simulink model "quietdriverMV"  (R2024b)
settings: Solver=VariableStepAuto  StartTime=0.0  StopTime=100  RelTol=1e-3
libraries: simulink x1
settings Model: Creator=sprinkle
settings OptimizationCC: ReuseModelBlockBuffer=off
settings RTWCC: GPUComputeCapability=3.5

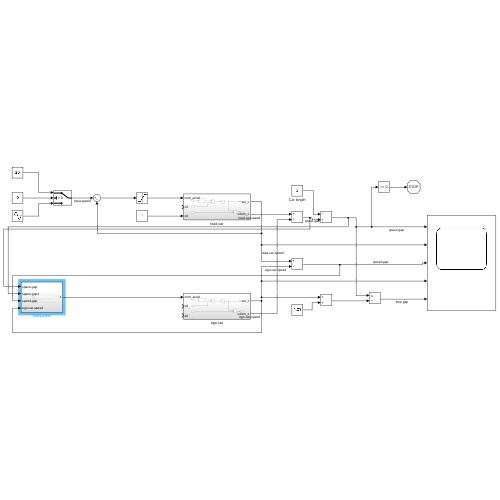
[thumbnail: Simulink's stored preview of the top-level diagram]
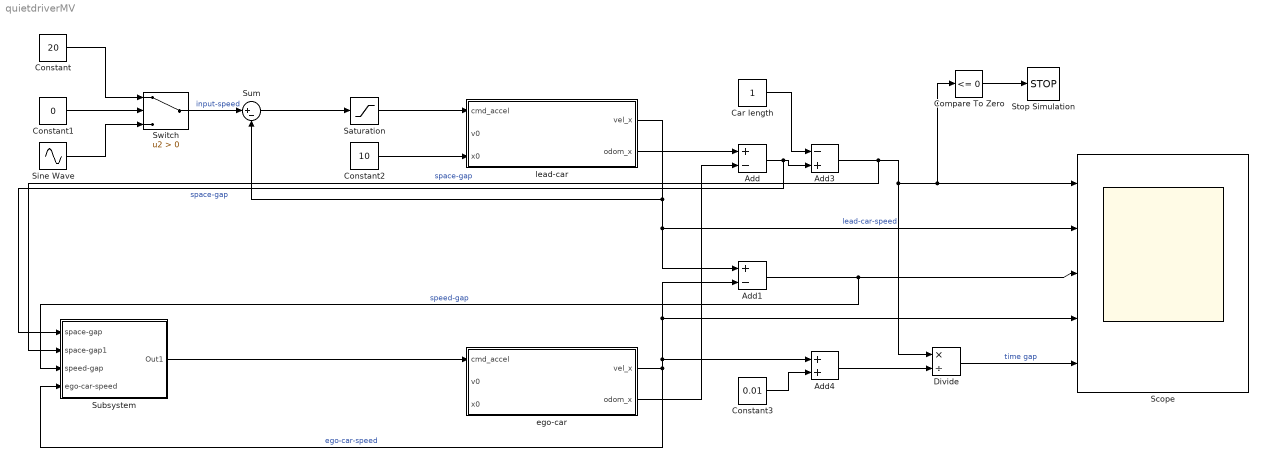
== system quietdriverMV ==
  Add : Sum  Inputs=+-
  Add1 : Sum  Inputs=+-
  Add3 : Sum  Inputs=-+
  Add4 : Sum
  Car length : Constant
  Compare To Zero : simulink/Logic and Bit Operations/Compare To Zero  relop=<=  OutDataTypeStr=boolean
  Constant : Constant  Value=20
  Constant1 : Constant  Value=0
  Constant2 : Constant  Value=10
  Constant3 : Constant  Value=0.01
  Divide : Product  Inputs=*/
  Saturation : Saturate  UpperLimit=1.5  LowerLimit=-3
  Scope : Scope  NumInputPorts=5
  Sine Wave : Sin  Bias=20  SampleTime=0
  Stop Simulation : Stop
  Subsystem : Subsystem
  Sum : Sum  Inputs=|+-
  Switch : Switch  Criteria=u2 > Threshold  SaturateOnIntegerOverflow=off  InputSameDT=off
  ego-car : Subsystem
  lead-car : Subsystem
  wires:
  Constant/1 -> Switch/1
  Sum/1 -> Saturation/1
  lead-car/1(vel_x) -> Add1/1, Scope/2, Sum/2  "lead-car-speed"
  Saturation/1 -> lead-car/1(cmd_accel)
  Switch/1 -> Sum/1  "input-speed"
  Sine Wave/1 -> Switch/3
  Constant1/1 -> Switch/2
  ego-car/1(vel_x) -> Subsystem/4(ego-car-speed), Add1/2, Scope/4, Add4/1  "ego-car-speed"
  lead-car/2(odom_x) -> Add/1
  ego-car/2(odom_x) -> Add/2
  Add3/1 -> Subsystem/2(space-gap1), Divide/1, Compare To Zero/1, Scope/1  "space-gap"
  Add1/1 -> Subsystem/3(speed-gap), Scope/3  "speed-gap"
  Constant2/1 -> lead-car/3(x0)
  Car length/1 -> Add3/1
  Add/1 -> Subsystem/1(space-gap), Add3/2  "space-gap"
  Divide/1 -> Scope/5  "time gap"
  Add4/1 -> Divide/2
  Constant3/1 -> Add4/2
  Compare To Zero/1 -> Stop Simulation/1
  Subsystem/1(Out1) -> ego-car/1(cmd_accel)

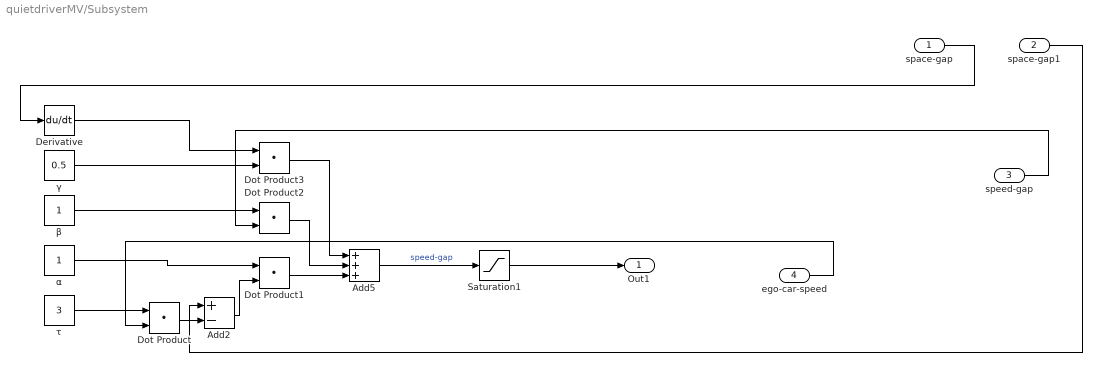
== system quietdriverMV/Subsystem ==
  space-gap : Inport
  space-gap1 : Inport  Port=2
  speed-gap : Inport  Port=3
  ego-car-speed : Inport  Port=4
  Add2 : Sum  Inputs=+-
  Add5 : Sum  Inputs=+++
  Derivative : Derivative
  Dot Product{,1..3} (4 alike) : DotProduct  OutDataTypeStr=Inherit: Inherit via internal rule
  Saturation1 : Saturate  UpperLimit=100  LowerLimit=-100
  α : Constant
  β : Constant
  γ : Constant  Value=0.5
  τ : Constant  Value=3
  Out1 : Outport
  wires:
  Dot Product/1 -> Add2/2
  α/1 -> Dot Product1/1
  space-gap1/1 -> Add2/1
  Add2/1 -> Dot Product1/2
  Saturation1/1 -> Out1/1
  Dot Product3/1 -> Add5/1
  β/1 -> Dot Product2/1
  Add5/1 -> Saturation1/1  "speed-gap"
  space-gap/1 -> Derivative/1
  Dot Product1/1 -> Add5/3
  γ/1 -> Dot Product3/2
  ego-car-speed/1 -> Dot Product/2
  speed-gap/1 -> Dot Product2/2
  Dot Product2/1 -> Add5/2
  τ/1 -> Dot Product/1
  Derivative/1 -> Dot Product3/1

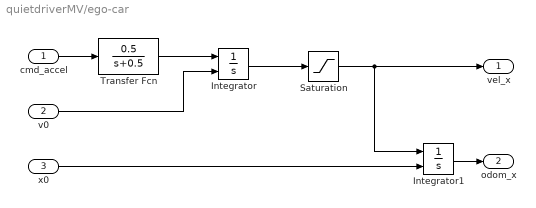
== system quietdriverMV/ego-car ==
  cmd_accel : Inport
  v0 : Inport  Port=2
  x0 : Inport  Port=3
  Integrator : Integrator  InitialConditionSource=external
  Integrator1 : Integrator  InitialConditionSource=external
  Saturation : Saturate  UpperLimit=80  LowerLimit=0
  Transfer Fcn : TransferFcn  Numerator=[0.5]  Denominator=[1 0.5]
  vel_x : Outport
  odom_x : Outport  Port=2
  wires:
  v0/1 -> Integrator/2
  cmd_accel/1 -> Transfer Fcn/1
  Transfer Fcn/1 -> Integrator/1
  Integrator1/1 -> odom_x/1
  Integrator/1 -> Saturation/1
  x0/1 -> Integrator1/2
  Saturation/1 -> vel_x/1, Integrator1/1

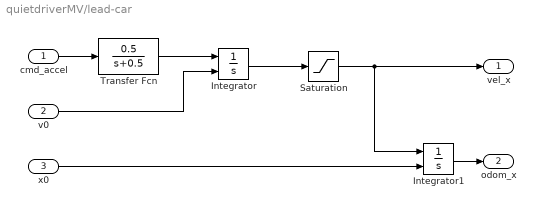
== system quietdriverMV/lead-car ==
  cmd_accel : Inport
  v0 : Inport  Port=2
  x0 : Inport  Port=3
  Integrator : Integrator  InitialConditionSource=external
  Integrator1 : Integrator  InitialConditionSource=external
  Saturation : Saturate  UpperLimit=80  LowerLimit=0
  Transfer Fcn : TransferFcn  Numerator=[0.5]  Denominator=[1 0.5]
  vel_x : Outport
  odom_x : Outport  Port=2
  wires:
  v0/1 -> Integrator/2
  cmd_accel/1 -> Transfer Fcn/1
  Transfer Fcn/1 -> Integrator/1
  Integrator1/1 -> odom_x/1
  Integrator/1 -> Saturation/1
  x0/1 -> Integrator1/2
  Saturation/1 -> vel_x/1, Integrator1/1
